simulink model "Feedback_DC_motor_model"  (R2017a)
settings: Solver=VariableStepAuto  StartTime=0.0  StopTime=10.0  RelTol=1e-3
values from neighbouring files (symbols this model uses):
  B = 9.55e-4    (= 0.000955)    [DCParams.m]
  J = 0.0038    [DCParams.m]
  Kt = 10.02    [DCParams.m]
  Kv = 0.0708    [DCParams.m]
  La = 3.39e-3    (= 0.00339)    [DCParams.m]
  Ra = 1.64    [DCParams.m]
  Tload = 0    [DCParams.m]
undefined symbols (not defined in the file or in its folder): K1, K2
settings Model: Creator=Merc  LastModifiedBy=Merc

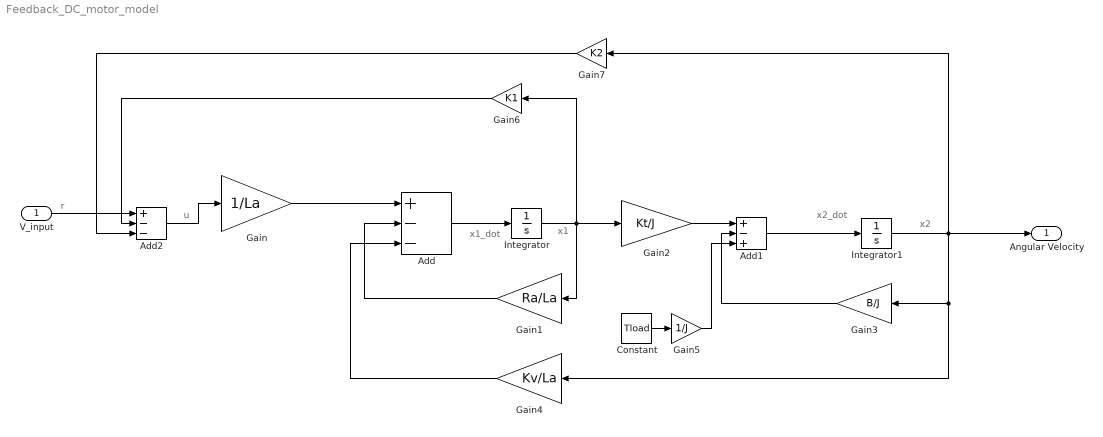
== system Feedback_DC_motor_model ==
  note: r
  note: u
  note: x2
  note: x2_dot
  note: x1
  note: x1_dot
  V_input : Inport
  Add : Sum  Inputs=+--
  Add1 : Sum  Inputs=+-+
  Add2 : Sum  Inputs=+--
  Constant : Constant  Value=Tload
  Gain : Gain  Gain=1/La
  Gain1 : Gain  Gain=Ra/La
  Gain2 : Gain  Gain=Kt/J
  Gain3 : Gain  Gain=B/J
  Gain4 : Gain  Gain=Kv/La
  Gain5 : Gain  Gain=1/J
  Gain6 : Gain  Gain=K1
  Gain7 : Gain  Gain=K2
  Integrator : Integrator  InitialCondition=1
  Integrator1 : Integrator  InitialCondition=1
  Angular Velocity : Outport
  wires:
  Gain/1 -> Add/1
  Add/1 -> Integrator/1
  Integrator/1 -> Gain6/1, Gain1/1, Gain2/1
  Gain1/1 -> Add/2
  Gain2/1 -> Add1/1
  Add1/1 -> Integrator1/1
  Integrator1/1 -> Gain7/1, Angular Velocity/1, Gain4/1, Gain3/1
  Gain3/1 -> Add1/2
  Gain4/1 -> Add/3
  Constant/1 -> Gain5/1
  Gain5/1 -> Add1/3
  V_input/1 -> Add2/1
  Add2/1 -> Gain/1
  Gain6/1 -> Add2/2
  Gain7/1 -> Add2/3
